simulink model "EV_SmartGrid"  (R2024a)
settings: Solver=FixedStepDiscrete  StartTime=0  StopTime=24  FixedStep=0.25  RelTol=1e-3
undefined symbols (not defined in the file or in its folder): DiscIntNeverNeededParam
settings Model: Creator=KrishanPC  LastModifiedBy=KrishanPC

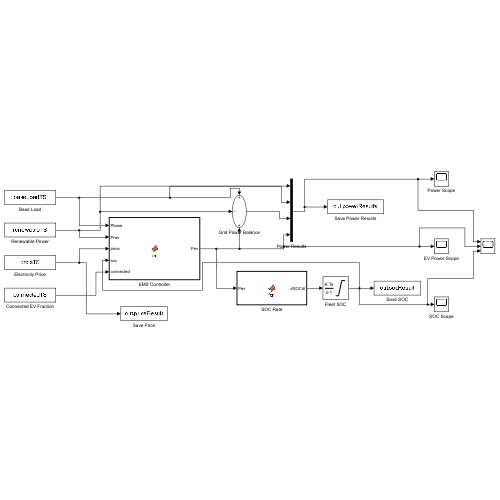
[thumbnail: Simulink's stored preview of the top-level diagram]
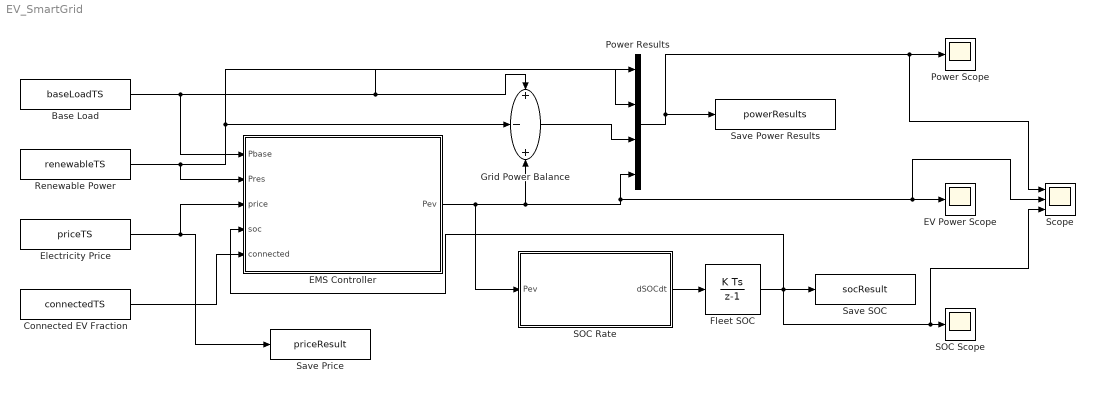
== system EV_SmartGrid ==
  Base Load : FromWorkspace  VariableName=baseLoadTS
  Connected EV Fraction : FromWorkspace  VariableName=connectedTS
  EMS Controller : MATLAB Function  TreatAsAtomicUnit=on
  EV Power Scope : Scope
  Electricity Price : FromWorkspace  VariableName=priceTS
  Fleet SOC : DiscreteIntegrator  InitialCondition=0.45  SampleTime=0.25  LimitOutput=on  UpperSaturationLimit=0.95  LowerSaturationLimit=0.20  ICPrevOutput=DiscIntNeverNeededParam  ICPrevScaledInput=DiscIntNeverNeededParam
  Grid Power Balance : Sum  Inputs=+-+
  Power Results : Mux
  Power Scope : Scope
  Renewable Power : FromWorkspace  VariableName=renewableTS
  SOC Rate : MATLAB Function  TreatAsAtomicUnit=on
  SOC Scope : Scope
  Save Power Results : ToWorkspace  VariableName=powerResults  SaveFormat=Timeseries  SampleTime=-1
  Save Price : ToWorkspace  VariableName=priceResult  SaveFormat=Timeseries  SampleTime=-1
  Save SOC : ToWorkspace  VariableName=socResult  SaveFormat=Timeseries  SampleTime=-1
  Scope : Scope  NumInputPorts=3
  wires:
  Base Load/1 -> Grid Power Balance/1, Power Results/1, EMS Controller/1(Pbase)
  Renewable Power/1 -> Grid Power Balance/2, Power Results/2, EMS Controller/2(Pres)
  Electricity Price/1 -> EMS Controller/3(price), Save Price/1
  Fleet SOC/1 -> EMS Controller/4(soc), Save SOC/1, Scope/3, SOC Scope/1
  Connected EV Fraction/1 -> EMS Controller/5(connected)
  EMS Controller/1(Pev) -> Grid Power Balance/3, Power Results/4, Scope/2, EV Power Scope/1, SOC Rate/1(Pev)
  SOC Rate/1(dSOCdt) -> Fleet SOC/1
  Grid Power Balance/1 -> Power Results/3
  Power Results/1 -> Power Scope/1, Scope/1, Save Power Results/1

== matlab function EV_SmartGrid/SOC Rate ==
  data: Pev input; dSOCdt output
function dSOCdt = fcn(Pev)

% Total energy capacity:
% 50 EVs multiplied by 60 kWh per EV

totalCapacity = 50*60;

chargeEfficiency = 0.94;
dischargeEfficiency = 0.92;

if Pev >= 0

    % Grid-to-vehicle charging
    dSOCdt = chargeEfficiency*Pev/totalCapacity;

else

    % Vehicle-to-grid discharging
    dSOCdt = Pev/(dischargeEfficiency*totalCapacity);

end

end

== matlab function EV_SmartGrid/EMS Controller ==
  data: Pbase input; Pev output; Pres input; price input; soc input; connected input
function Pev = fcn(Pbase, Pres, price, soc, connected)

% Pev > 0: EV charging
% Pev < 0: V2G discharging

%% Fleet limits

connected = min(max(connected,0),1);

maxCharge = 360*connected;
maxDischarge = 250*connected;

transformerLimit = 500;

%% Grid power before EV charging

netWithoutEV = Pbase - Pres;

%% Charging decision

if connected < 0.02

    % Almost no EVs are connected
    Pev = 0;

elseif soc <= 0.23

    % SOC is low, so charging has priority
    Pev = maxCharge;

elseif Pres > Pbase && soc < 0.90

    % Use surplus renewable energy
    Pev = min(maxCharge,Pres-Pbase);

elseif price <= 0.11 && soc < 0.80

    % Charge during low-price periods
    Pev = 0.75*maxCharge;

elseif netWithoutEV >= 390 && soc > 0.55

    % Discharge to reduce the grid peak
    Pev = -min(maxDischarge,netWithoutEV-350);

elseif price >= 0.28 && soc > 0.60

    % V2G during expensive periods
    Pev = -0.45*maxDischarge;

elseif soc < 0.65

    % Slow background charging
    Pev = 0.25*maxCharge;

else

    Pev = 0;

end

%% Charger power limits

Pev = min(Pev,maxCharge);
Pev = max(Pev,-maxDischarge);

%% Transformer import limit

availablePower = transformerLimit-netWithoutEV;
Pev = min(Pev,availablePower);

%% Final battery safety

if soc <= 0.20 && Pev < 0
    Pev = 0;
end

if soc >= 0.95 && Pev > 0
    Pev = 0;
end

end
